simulink model "ready_to_copy_for_lab"  (R2023b)
settings: Solver=VariableStepAuto  StartTime=0.0  StopTime=10.0  RelTol=1e-3
values from neighbouring files (symbols this model uses):
  A = double(A)    [consistent.m]    (also in dyn_model_mark.m)
  B = double(B)    [consistent.m]    (also in dyn_model_mark.m)
  x1_bar = 0    [consistent.m]    (also in dyn_model_mark.m)
  x3_bar = 0    [consistent.m]    (also in dyn_model_mark.m = 3.14159265359)
undefined symbols (not defined in the file or in its folder): A_uns, B_uns, K_lq, K_lq_uns, x1_bar_uns, x3_bar_uns
libraries: simulink_extras x7, simulink x1
settings Model: Creator=Mark  LastModifiedBy=Mark

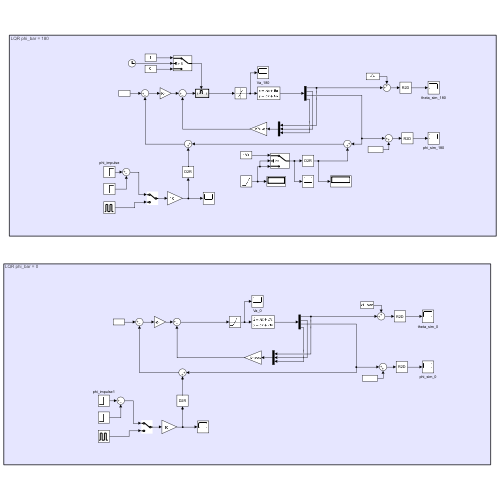
[thumbnail: Simulink's stored preview of the top-level diagram]
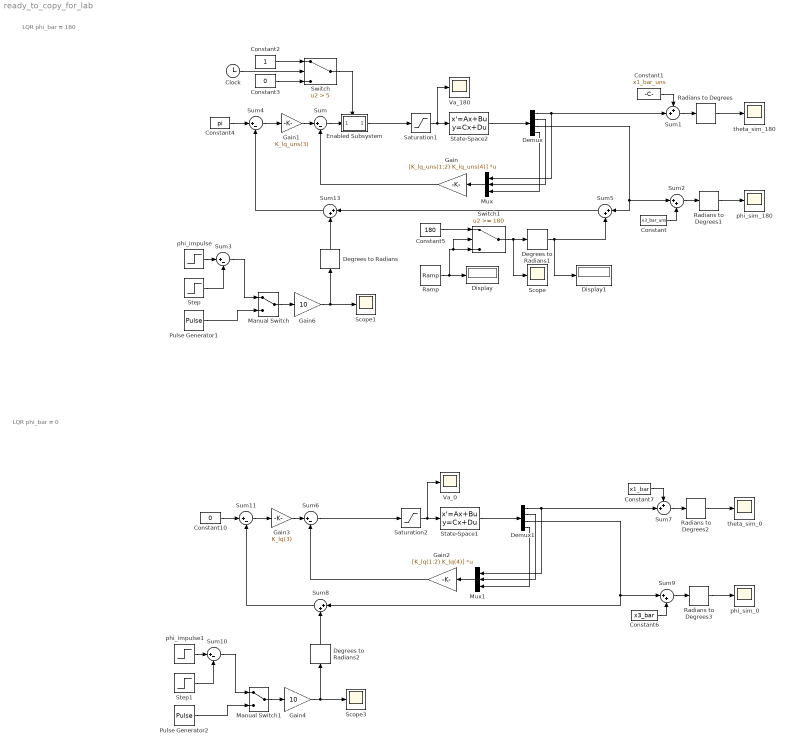
== system ready_to_copy_for_lab ==
  note: LQR phi_bar = 0
  note: LQR phi_bar = 180
  Clock : Clock
  Constant : Constant  Value=x3_bar_uns
  Constant1 : Constant  Value=x1_bar_uns
  Constant10 : Constant  Value=0
  Constant2 : Constant
  Constant3 : Constant  Value=0
  Constant4 : Constant  Value=pi
  Constant5 : Constant  Value=180
  Constant6 : Constant  Value=x3_bar
  Constant7 : Constant  Value=x1_bar
  Degrees to Radians : simulink_extras/Transformations/Degrees to Radians
  Degrees to Radians1 : simulink_extras/Transformations/Degrees to Radians
  Degrees to Radians2 : simulink_extras/Transformations/Degrees to Radians
  Demux : Demux
  Demux1 : Demux
  Display : Display
  Display1 : Display
  Enabled Subsystem : Subsystem  TreatAsAtomicUnit=on
  Gain : Gain  Gain=[K_lq_uns(1:2) K_lq_uns(4)]  Multiplication=Matrix(K*u) (u vector)
  Gain1 : Gain  Gain=K_lq_uns(3)
  Gain2 : Gain  Gain=[K_lq(1:2) K_lq(4)]  Multiplication=Matrix(K*u) (u vector)
  Gain3 : Gain  Gain=K_lq(3)
  Gain4 : Gain  Gain=10
  Gain6 : Gain  Gain=10
  Manual Switch : ManualSwitch
  Manual Switch1 : ManualSwitch
  Mux : Mux  Inputs=3
  Mux1 : Mux  Inputs=3
  Pulse Generator1 : DiscretePulseGenerator  PulseType=Time based  Period=4  PulseWidth=50  PhaseDelay=10
  Pulse Generator2 : DiscretePulseGenerator  PulseType=Time based  Period=4  PulseWidth=50  PhaseDelay=10
  Radians to Degrees{,1..3} (4 alike) : simulink_extras/Transformations/Radians to Degrees
  Ramp : simulink/Sources/Ramp  slope=50  start=0  InitialOutput=0
  Saturation1 : Saturate  UpperLimit=10  LowerLimit=-10
  Saturation2 : Saturate  UpperLimit=10  LowerLimit=-10
  Scope : Scope
  Scope1 : Scope
  Scope3 : Scope
  State-Space1 : StateSpace  A=A  B=B  C=eye(4)  D=zeros(4,1)  InitialCondition=[0 0 0 0]
  State-Space2 : StateSpace  A=A_uns  B=B_uns  C=eye(4)  D=zeros(4,1)  InitialCondition=[0 0 0 0]
  Step : Step  Time=30.5  SampleTime=0
  Step1 : Step  Time=30.5  SampleTime=0
  Sum{,3..4,6,10..11} (6 alike) : Sum  Inputs=|+-
  Sum1 : Sum  Inputs=++|
  Sum{2,5,8..9,13} (5 alike) : Sum  Inputs=|++
  Sum7 : Sum  Inputs=++|
  Switch : Switch  Criteria=u2 > Threshold  Threshold=5  SaturateOnIntegerOverflow=off  InputSameDT=off
  Switch1 : Switch  Threshold=180  SaturateOnIntegerOverflow=off  InputSameDT=off
  Va_0 : Scope
  Va_180 : Scope
  phi_impulse : Step  Time=30  SampleTime=0
  phi_impulse1 : Step  Time=30  SampleTime=0
  phi_sim_0 : Scope
  phi_sim_180 : Scope
  theta_sim_0 : Scope
  theta_sim_180 : Scope
  wires:
  Enabled Subsystem/1(Out1) -> Saturation1/1
  Constant2/1 -> Switch/1
  Constant3/1 -> Switch/3
  Constant4/1 -> Sum4/1
  Sum5/1 -> Sum13/1
  Degrees to Radians1/1 -> Sum5/2, Display1/1
  Switch/1 -> Enabled Subsystem/Enable
  Constant5/1 -> Switch1/1
  Gain2/1 -> Sum6/2
  Mux1/1 -> Gain2/1
  Constant6/1 -> Sum9/2
  Sum10/1 -> Manual Switch1/1
  Radians to Degrees3/1 -> phi_sim_0/1
  phi_impulse1/1 -> Sum10/1
  Sum9/1 -> Radians to Degrees3/1
  Step1/1 -> Sum10/2
  Pulse Generator2/1 -> Manual Switch1/2
  Saturation2/1 -> Va_0/1, State-Space1/1
  Radians to Degrees2/1 -> theta_sim_0/1
  Degrees to Radians2/1 -> Sum8/2
  Demux1/1 -> Sum7/2, Mux1/1
  Constant7/1 -> Sum7/1
  Sum11/1 -> Gain3/1
  Manual Switch1/1 -> Gain4/1
  State-Space1/1 -> Demux1/1
  Sum8/1 -> Sum11/2
  Constant10/1 -> Sum11/1
  Manual Switch/1 -> Gain6/1
  State-Space2/1 -> Demux/1
  Demux/3 -> Sum5/1, Sum2/1
  Clock/1 -> Switch/2
  Sum13/1 -> Sum4/2
  Gain1/1 -> Sum/1
  Sum1/1 -> Radians to Degrees/1
  Demux1/3 -> Sum8/1, Sum9/1
  Constant1/1 -> Sum1/1
  Demux/1 -> Sum1/2, Mux/1
  Sum4/1 -> Gain1/1
  Degrees to Radians/1 -> Sum13/2
  Gain3/1 -> Sum6/1
  Saturation1/1 -> Va_180/1, State-Space2/1
  Gain4/1 -> Scope3/1, Degrees to Radians2/1
  Demux/4 -> Mux/3
  Demux1/2 -> Mux1/2
  Radians to Degrees/1 -> theta_sim_180/1
  Sum/1 -> Enabled Subsystem/1(In1)
  Demux/2 -> Mux/2
  Gain6/1 -> Scope1/1, Degrees to Radians/1
  Sum2/1 -> Radians to Degrees1/1
  Pulse Generator1/1 -> Manual Switch/2
  phi_impulse/1 -> Sum3/1
  Sum3/1 -> Manual Switch/1
  Constant/1 -> Sum2/2
  Demux1/4 -> Mux1/3
  Sum6/1 -> Saturation2/1
  Step/1 -> Sum3/2
  Sum7/1 -> Radians to Degrees2/1
  Switch1/1 -> Scope/1, Degrees to Radians1/1
  Radians to Degrees1/1 -> phi_sim_180/1
  Ramp/1 -> Switch1/2, Switch1/3, Display/1
  Gain/1 -> Sum/2
  Mux/1 -> Gain/1

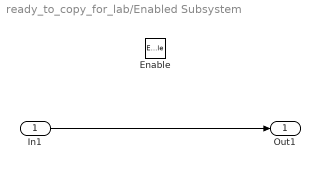
== system ready_to_copy_for_lab/Enabled Subsystem ==
  In1 : Inport
  Enable : EnablePort
  Out1 : Outport
  wires:
  In1/1 -> Out1/1
